simulink model "db_ej_engranes"  (R2020b)
settings: Solver=VariableStepAuto  StartTime=0.0  StopTime=40  RelTol=1e-3
undefined symbols (not defined in the file): A, B, B1, B2, C, D, J1, J2, K1, K2, r1, r2, u1, u2
settings Model: Creator=carma  LastModifiedBy=carma
settings DataIOCC: ReturnWorkspaceOutputs=off
settings DebuggingCC: ArithmeticOperatorsInVariantConditions=warning
settings SFSimCC: SimUseLocalCustomCode=off  CustomCodeUndefinedFunction=UseInterfaceOnly
settings RTWCC: RTWUseLocalCustomCode=off

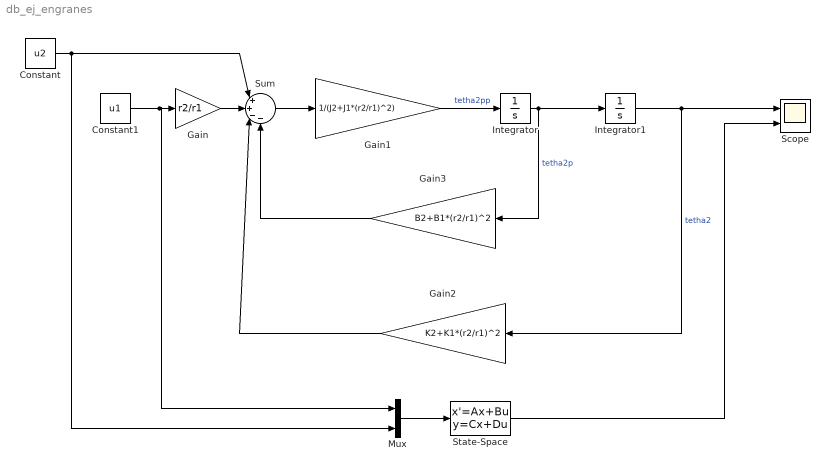
== system db_ej_engranes ==
  Constant : Constant  Value=u2
  Constant1 : Constant  Value=u1
  Gain : Gain  Gain=r2/r1
  Gain1 : Gain  Gain=1/(J2+J1*(r2/r1)^2)
  Gain2 : Gain  Gain=K2+K1*(r2/r1)^2
  Gain3 : Gain  Gain=B2+B1*(r2/r1)^2
  Integrator : Integrator
  Integrator1 : Integrator
  Mux : Mux  Inputs=2
  Scope : Scope  NumInputPorts=2
  State-Space : StateSpace  A=A  B=B  C=C  D=D  InitialCondition=0
  Sum : Sum  Inputs=|++--
  wires:
  Constant/1 -> Mux/2, Sum/1
  Gain/1 -> Sum/2
  Constant1/1 -> Mux/1, Gain/1
  Sum/1 -> Gain1/1
  Gain1/1 -> Integrator/1  "tetha2pp"
  Integrator/1 -> Gain3/1, Integrator1/1  "tetha2p"
  Integrator1/1 -> Gain2/1, Scope/1  "tetha2"
  Gain2/1 -> Sum/3
  Gain3/1 -> Sum/4
  Mux/1 -> State-Space/1
  State-Space/1 -> Scope/2
